simulink model "Model_1_AMBD"  (R2025b)
settings: Solver=VariableStepAuto  StartTime=0.0  StopTime=25  RelTol=1e-3
libraries: autolibshared x3
(part 3 of 3)

== stateflow chart Model_1_AMBD/Subsystem/Conroller ==
  state Idle
    en: Demand_Torque = 0;
  state Braking
    en: Demand_Torque = -1200;
  state Accelerating
    en: Demand_Torque = Max_Torque;
  state Cruising
    en: Demand_Torque = 80;
  (default) -> Idle
  Braking -> Idle : [after(5, sec)]
  Idle -> Accelerating : [after(5, sec)]
  Accelerating -> Cruising : [after(5, sec)]
  Cruising -> Braking : [after(5, sec)]
  data: Max_Torque input; Throttle input; Demand_Torque output
